simulink model "CAR_CONTROL_SYSTEM"  (R2024b)
settings: Solver=FixedStepAuto  StartTime=0.0  StopTime=inf  FixedStep=1e-3  RelTol=1e-3  EnableMultiTasking=on
model workspace (MAT data in the model file):
  SL_ROS_VariableLengthArrays_MaxSizes : object (value not decoded)
undefined symbols (not defined in the file or in its folder): angular, CIRCUIT, CLTF_DAMP, CLTF_FREQ, CLTF_GAIN, CONTROL, CONTROL_INI, DiscIntNeverNeededParam, dspblkCoreblockFVToolHelper, gcbh, INPUT, linear, MCP3201, MD25, MODEL, MODEL_INI, mpcstate, MPU60X0, MPU9250, MSG, NAV_MPC_CONTROL, OUTPUT, SAMPLING_TIME, SYSID_INPUT, VL6180X
libraries: raspberrypiCommlib x153, simulink x85, raspberrypiNetworklib x8, embedlinuxBasiclib x6, ctrlSharedLib x2, ros2lib x2, mpclib x1, vrlib x1, sldrtlib x1
(part 2 of 16)

== system CAR_CONTROL_SYSTEM/HARDWARE/COMMUNICATIONS ==
  MCS_RX : Subsystem  Commented=on  TreatAsAtomicUnit=on
      settings: MinAlgLoopOccurrences=on
  TCP/IP : Subsystem  TreatAsAtomicUnit=on
      settings: MinAlgLoopOccurrences=on
  TCP/IP RPI4 : Subsystem  TreatAsAtomicUnit=on
      settings: MinAlgLoopOccurrences=on

== system CAR_CONTROL_SYSTEM/HARDWARE/SENSORS ==
  BUTTONS : Subsystem  TreatAsAtomicUnit=on
      settings: MinAlgLoopOccurrences=on
  CURRENT_ADC_MCP3201_SPI : Subsystem  Commented=on  TreatAsAtomicUnit=on
      settings: RTWSystemCode=Nonreusable function  FunctionWithSeparateData=on
  IMU MPU60X0_SPI : Subsystem  Priority=0  TreatAsAtomicUnit=on
      settings: MinAlgLoopOccurrences=on  RTWSystemCode=Nonreusable function  FunctionWithSeparateData=on
  RCRX iBUS : Subsystem  TreatAsAtomicUnit=on
      settings: MinAlgLoopOccurrences=on
  WALL RANGE SENSOR : Subsystem
      settings: MinAlgLoopOccurrences=on

== system CAR_CONTROL_SYSTEM/MONITORING/BLACKBOX ==
  Compare To Constant : simulink/Logic and Bit Operations/Compare To Constant  relop===  const=uint8(2)  OutDataTypeStr=boolean
  Compare To Constant1 : simulink/Logic and Bit Operations/Compare To Constant  relop=>  const=uint8(2)  OutDataTypeStr=boolean
  Compare To Constant2 : simulink/Logic and Bit Operations/Compare To Constant  relop=~=  const=uint8(11)  OutDataTypeStr=boolean
  Data Store Read9 : DataStoreRead  DataStoreName=CONTROL  SampleTime=SAMPLING_TIME  DataStoreElements=CONTROL.STATE.COMM_MODE#CONTROL.STATE.CURRENT_STATUS_SYS  IndexOptions=Index vector (dialog)  Indices=1  OutputSizes=1
  HARDWARE: BLACKBOX : Subsystem  Priority=1000
  Logical Operator : Logic  Inputs=3  AllPortsSameDT=off  OutDataTypeStr=boolean
  PC: BLACKBOX : Subsystem
  wires:
  Data Store Read9/1 -> Compare To Constant/1
  Data Store Read9/2 -> Compare To Constant2/1, Compare To Constant1/1
  Compare To Constant/1 -> Logical Operator/1
  Compare To Constant1/1 -> Logical Operator/2
  Compare To Constant2/1 -> Logical Operator/3
  Logical Operator/1 -> HARDWARE: BLACKBOX/Enable, PC: BLACKBOX/Enable

== system CAR_CONTROL_SYSTEM/MONITORING/COMMUNICATIONS ==
  Compare To Zero1 : simulink/Logic and Bit Operations/Compare To Zero  relop=>  OutDataTypeStr=boolean
  Compare To Zero2 : simulink/Logic and Bit Operations/Compare To Zero  relop=>  OutDataTypeStr=boolean
  Data Store Read1 : DataStoreRead  DataStoreName=MSG  SampleTime=CONTROL_INI.PARAM.COMM_SAMPLING_TIME  DataStoreElements=MSG.RX_BUFFER(1,1)  IndexOptions=Index vector (dialog)  Indices=1  OutputSizes=1
  Data Store Read3 : DataStoreRead  DataStoreName=MSG  SampleTime=CONTROL_INI.PARAM.COMM_SAMPLING_TIME  DataStoreElements=MSG.TX_ID(1,1)  IndexOptions=Index vector (dialog)  Indices=1  OutputSizes=1
  MSG_RX : Subsystem  Priority=10
      settings: RTWSystemCode=Nonreusable function  FunctionWithSeparateData=on
  "MSG_TX " : Subsystem  Priority=10
      settings: RTWSystemCode=Nonreusable function  FunctionWithSeparateData=on
  wires:
  Data Store Read3/1 -> Compare To Zero2/1
  Compare To Zero2/1 -> "MSG_TX "/Enable
  Data Store Read1/1 -> Compare To Zero1/1
  Compare To Zero1/1 -> MSG_RX/Enable

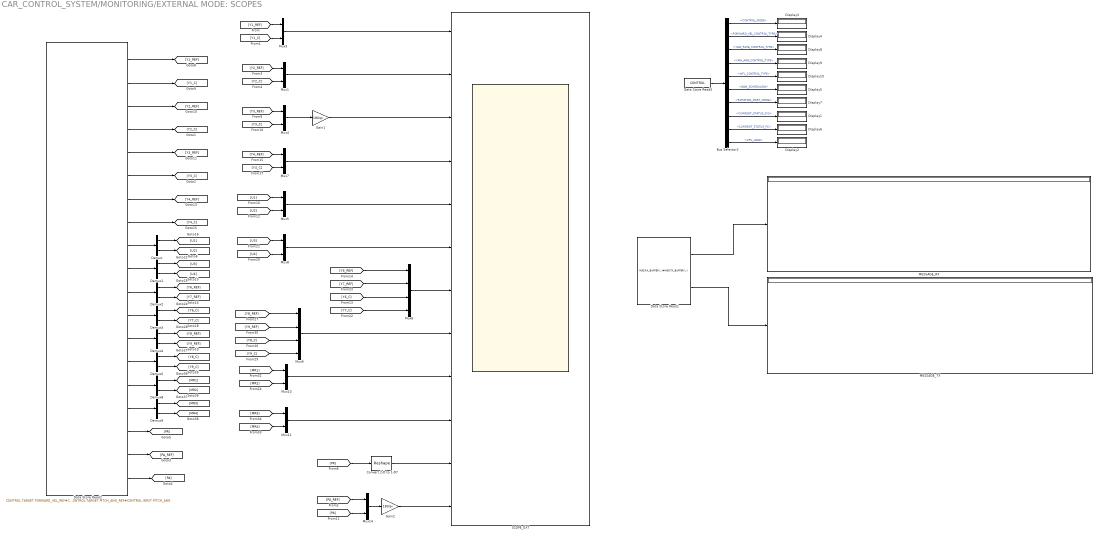
== system CAR_CONTROL_SYSTEM/MONITORING/EXTERNAL MODE: SCOPES ==
  Bus Selector2 : BusSelector  OutputSignals=STATE.CONTROL_MODE,STATE.FORWARD_VEL_CONTROL_TYPE,STATE.YAW_RATE_CONTROL_TYPE,STATE.YAW_ANG_CONTROL_TYPE,STATE.WFL_CONTROL_TYPE,STATE.GAIN_SCHEDULING,STATE.ROTATION_MSRT_MODE,STATE.CURRENT_STATUS_SYS,STATE.CURRENT_STATUS_PC,STATE.CPU_LOAD
  Convert 2-D to 1-D7 : Reshape
  Data Store Read1 : DataStoreRead  DataStoreName=MSG  SampleTime=SAMPLING_TIME  DataStoreElements=MSG.RX_BUFFER(:,:)#MSG.TX_BUFFER(:,:)  IndexOptions=Index vector (dialog)  Indices=1  OutputSizes=1
  Data Store Read2 : DataStoreRead  DataStoreName=CONTROL  SampleTime=SAMPLING_TIME  DataStoreElements=CONTROL.TARGET.FORWARD_VEL_REF#CONTROL.INPUT.FORWARD_VEL#CONTROL.TARGET.YAW_RATE_REF#CONTROL.INPUT.YAW_RATE#CONTROL.TARGET.YAW_ANG_REF#CONTROL.INPUT.YAW_ANG#CONTROL.TARGET.WALL_DIST_REF#CONTROL.INPUT.WALL_DIST#CONTROL.OUTPUT.MOTOR_VOLT(:,:)#CONTROL.OUTPUT.MOTOR_VOLT_CD(:,:)#CONTROL.TARGET.POS_XY_REF(:,:)#CONTROL.INPUT.EARTH_POS(1:2,1)#CONTROL.TARGET.VEL_XY_REF(:,:)#CONTROL.INPUT.EARTH_VEL(1:2,1)#CONTROL.INPUT.MOTOR_RATE(:,:)#CONTROL.INPUT.MOTOR_RATE_CD(:,:)#CONTROL.INPUT.PITCH_RATE#CONTROL.TARGET.PITCH_ANG_REF#CONTROL.INPUT.PITCH_ANG  IndexOptions=Index vector (dialog)  Indices=1  OutputSizes=1
  Data Store Read5 : DataStoreRead  DataStoreName=CONTROL  SampleTime=SAMPLING_TIME  IndexOptions=Index vector (dialog)  Indices=1  OutputSizes=1
  Demux{,1..5,8..9} (8 alike) : Demux  Outputs=2
  Display{1..10} (10 alike) : Display
  Gain1 : Gain  Gain=180/pi
  Gain2 : Gain  Gain=180/pi
  MESSAGE_RX : Display
  MESSAGE_TX : Display
  Mux{1,3..5,7..8,10..11,14} (9 alike) : Mux  Inputs=2
  Mux6 : Mux
  Mux9 : Mux
  SCOPE_EXT : Scope  NumInputPorts=12
  wires:
  Data Store Read5/1 -> Bus Selector2/1
  Bus Selector2/7 -> Display7/1  "<ROTATION_MSRT_MODE>"
  Data Store Read1/1 -> MESSAGE_RX/1
  Bus Selector2/2 -> Display4/1  "<FORWARD_VEL_CONTROL_TYPE>"
  Bus Selector2/1 -> Display3/1  "<CONTROL_MODE>"
  Bus Selector2/6 -> Display5/1  "<GAIN_SCHEDULING>"
  Bus Selector2/8 -> Display1/1  "<CURRENT_STATUS_SYS>"
  Bus Selector2/10 -> Display2/1  "<CPU_LOAD>"
  Data Store Read1/2 -> MESSAGE_TX/1
  Bus Selector2/9 -> Display6/1  "<CURRENT_STATUS_PC>"
  Demux8/2 -> [MR2]
  Demux9/1 -> [MR3]
  Data Store Read2/16 -> Demux9/1
  Data Store Read2/15 -> Demux8/1
  Data Store Read2/2 -> [Y1_C]
  Data Store Read2/7 -> [Y4_REF]
  Demux4/1 -> [Y8_REF]
  Demux5/1 -> [Y8_C]
  Demux3/1 -> [Y6_C]
  Demux2/1 -> [Y6_REF]
  Demux1/1 -> [U3]
  Demux3/2 -> [Y7_C]
  Demux5/2 -> [Y9_C]
  Demux4/2 -> [Y9_REF]
  Demux2/2 -> [Y7_REF]
  Data Store Read2/5 -> [Y3_REF]
  Demux/2 -> [U2]
  Data Store Read2/1 -> [Y1_REF]
  Demux1/2 -> [U4]
  Demux8/1 -> [MR1]
  Data Store Read2/4 -> [Y2_C]
  Data Store Read2/6 -> [Y3_C]
  Demux9/2 -> [MR4]
  Data Store Read2/3 -> [Y2_REF]
  Data Store Read2/8 -> [Y4_C]
  Demux/1 -> [U1]
  [MR1] -> Mux10/1
  [MR4] -> Mux11/2
  Gain1/1 -> SCOPE_EXT/3
  Mux10/1 -> SCOPE_EXT/9
  Mux8/1 -> SCOPE_EXT/6
  Mux6/1 -> SCOPE_EXT/7
  Mux5/1 -> SCOPE_EXT/5
  Mux7/1 -> SCOPE_EXT/4
  [MR3] -> Mux11/1
  [U4] -> Mux8/2
  Mux11/1 -> SCOPE_EXT/10
  [Y8_REF] -> Mux9/1
  [Y4_REF] -> Mux7/1
  [Y3_C] -> Mux4/2
  [Y4_C] -> Mux7/2
  [U1] -> Mux5/1
  Mux9/1 -> SCOPE_EXT/8
  [Y1_C] -> Mux3/2
  [U3] -> Mux8/1
  [U2] -> Mux5/2
  [Y2_C] -> Mux1/2
  [Y2_REF] -> Mux1/1
  Mux3/1 -> SCOPE_EXT/1
  [Y1_REF] -> Mux3/1
  [MR2] -> Mux10/2
  Mux4/1 -> Gain1/1
  Mux1/1 -> SCOPE_EXT/2
  [Y3_REF] -> Mux4/1
  [Y6_REF] -> Mux6/1
  [Y9_C] -> Mux9/4
  [Y7_C] -> Mux6/4
  Data Store Read2/9 -> Demux/1
  Data Store Read2/10 -> Demux1/1
  Data Store Read2/11 -> Demux2/1
  Data Store Read2/12 -> Demux3/1
  Data Store Read2/13 -> Demux4/1
  Data Store Read2/14 -> Demux5/1
  Bus Selector2/3 -> Display8/1  "<YAW_RATE_CONTROL_TYPE>"
  Bus Selector2/4 -> Display9/1  "<YAW_ANG_CONTROL_TYPE>"
  Bus Selector2/5 -> Display10/1  "<WFL_CONTROL_TYPE>"
  Data Store Read2/19 -> [PA]
  Data Store Read2/18 -> [PA_REF]
  Data Store Read2/17 -> [PR]
  [PA_REF] -> Mux14/1
  [PA] -> Mux14/2
  Mux14/1 -> Gain2/1
  Gain2/1 -> SCOPE_EXT/12
  [PR] -> Convert 2-D to 1-D7/1
  [Y6_C] -> Mux6/3
  [Y7_REF] -> Mux6/2
  [Y9_REF] -> Mux9/2
  [Y8_C] -> Mux9/3
  Convert 2-D to 1-D7/1 -> SCOPE_EXT/11

== system CAR_CONTROL_SYSTEM/MONITORING/FV COMPETITION: SCOPES ==
  Data Store Read1 : DataStoreRead  DataStoreName=CONTROL  SampleTime=SAMPLING_TIME  DataStoreElements=CONTROL.TARGET.FORWARD_VEL_REF#CONTROL.INPUT.FORWARD_VEL#CONTROL.OUTPUT.MOTOR_VOLT_CD(1,1)#CONTROL.STATE.COMP_IAE  IndexOptions=Index vector (dialog)  Indices=1  OutputSizes=1
  Display : Display
  FV COMPETITION SCOPE: SIM : Scope  NumInputPorts=3
  Mux6 : Mux  Inputs=2
  wires:
  Mux6/1 -> FV COMPETITION SCOPE: SIM/1
  Data Store Read1/1 -> Mux6/1
  Data Store Read1/2 -> Mux6/2
  Data Store Read1/3 -> FV COMPETITION SCOPE: SIM/2
  Data Store Read1/4 -> Display/1, FV COMPETITION SCOPE: SIM/3

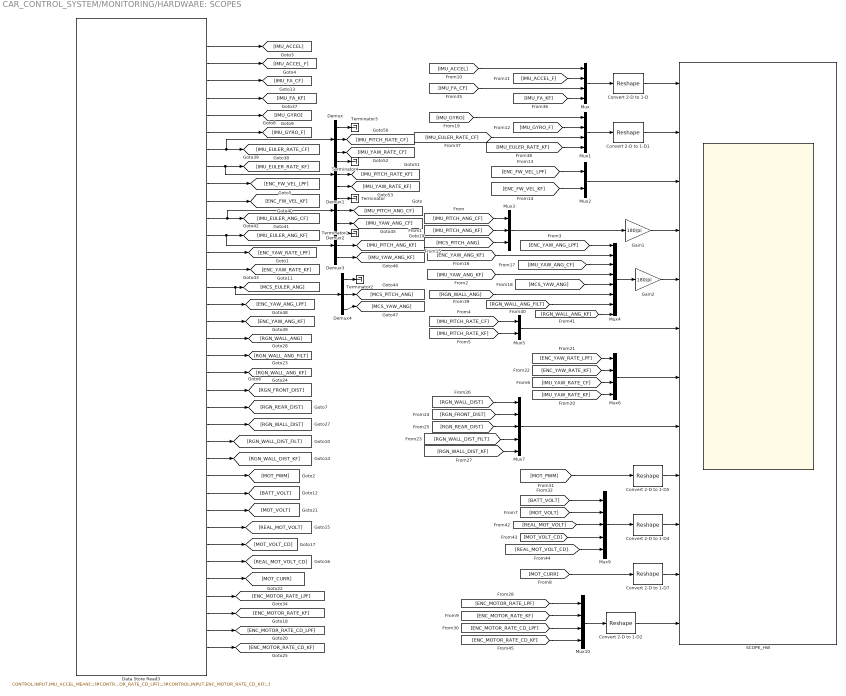
== system CAR_CONTROL_SYSTEM/MONITORING/HARDWARE: SCOPES ==
  Convert 2-D to 1-D{,1..2,4..5,7} (6 alike) : Reshape
  Data Store Read3 : DataStoreRead  DataStoreName=CONTROL  SampleTime=SAMPLING_TIME  DataStoreElements=CONTROL.INPUT.IMU_ACCEL_MEAN(:,:)#CONTROL.INPUT.IMU_ACCEL_MEAN_FILT(:,:)#CONTROL.INPUT.IMU_FORWARD_ACCEL_CF#CONTROL.INPUT.IMU_FORWARD_ACCEL_KF#CONTROL.INPUT.IMU_GYRO_MEAN(:,:)#CONTROL.INPUT.IMU_GYRO_MEAN_FILT(:,:)#CONTROL.INPUT.IMU_EULER_RATE_CF(:,:)#CONTROL.INPUT.IMU_EULER_RATE_KF(:,:)#CONTROL.INPUT.ENC_FORWARD_VEL_LPF#CONTROL.INPUT.ENC_FORWARD_VEL_KF#CONTROL.INPUT.IMU_EULER_ANG_CF(:,:)#CONTROL.INPUT.IMU_EULER_ANG_KF(:,:)#CONTROL.INPUT.ENC_YAW_RATE_LPF#CONTROL.INPUT.ENC_YAW_RATE_KF#CONTROL.INPUT.MCS_EULER_ANG(:,:)#CONTROL.INPUT.ENC_YAW_ANG_LPF#CONTROL.INPUT.ENC_YAW_ANG_KF#CONTROL.INPUT.RANGE_WALL_ANG#CONTROL.INPUT.WALL_ANG_FILT#CONTROL.INPUT.WALL_ANG_KF#CONTROL.INPUT.RANGE_FRONT_DIST#CONTROL.INPUT.RANGE_REAR_DIST#CONTROL.INPUT.RANGE_WALL_DIST#CONTROL.INPUT.WALL_DIST_FILT#CONTROL.INPUT.WALL_DIST_KF#CONTROL.OUTPUT.MOTOR_PWM(:,:)#CONTROL.INPUT.BATTERY_VOLT#CONTROL.OUTPUT.MOTOR_VOLT(:,:)#CONTROL.OUTPUT.REAL_MOTOR_VOLT(:,:)#CONTROL.OUTPUT.MOTOR_VOLT_CD(:,:)#CONTROL.OUTPUT.REAL_MOTOR_VOLT_CD(:,:)#CONTROL.INPUT.MOTOR_CURRENT(:,:)#CONTROL.INPUT.ENC_MOTOR_RATE_LPF(:,:)#CONTROL.INPUT.ENC_MOTOR_RATE_KF(:,:)#CONTROL.INPUT.ENC_MOTOR_RATE_CD_LPF(:,:)#CONTROL.INPUT.ENC_MOTOR_RATE_CD_KF(:,:)  IndexOptions=Index vector (dialog)  Indices=1  OutputSizes=1
  Demux{,1..4} (5 alike) : Demux  Outputs=3
  Gain1 : Gain  Gain=180/pi
  Gain2 : Gain  Gain=180/pi
  Mux{,1,6,10} (4 alike) : Mux
  Mux2 : Mux  Inputs=2
  Mux3 : Mux  Inputs=3
  Mux4 : Mux  Inputs=8
  Mux5 : Mux  Inputs=2
  Mux7 : Mux  Inputs=5
  Mux9 : Mux  Inputs=5
  SCOPE_HW : Scope  NumInputPorts=12
  Terminator{,1..4} (5 alike) : Terminator
  wires:
  [MOT_CURR] -> Convert 2-D to 1-D7/1
  Convert 2-D to 1-D/1 -> SCOPE_HW/1
  Convert 2-D to 1-D1/1 -> SCOPE_HW/2
  Mux2/1 -> SCOPE_HW/3
  [IMU_ACCEL] -> Mux/1
  Mux/1 -> Convert 2-D to 1-D/1
  [IMU_ACCEL_F] -> Mux/2
  [ENC_FW_VEL_LPF] -> Mux2/1
  [ENC_FW_VEL_KF] -> Mux2/2
  [IMU_PITCH_ANG_CF] -> Mux3/1
  [IMU_PITCH_ANG_KF] -> Mux3/2
  Mux3/1 -> Gain1/1
  Gain1/1 -> SCOPE_HW/4
  Mux4/1 -> Gain2/1
  Gain2/1 -> SCOPE_HW/5
  Mux5/1 -> SCOPE_HW/6
  [IMU_PITCH_RATE_CF] -> Mux5/1
  [IMU_PITCH_RATE_KF] -> Mux5/2
  Mux6/1 -> SCOPE_HW/7
  Mux7/1 -> SCOPE_HW/8
  [RGN_WALL_DIST] -> Mux7/1
  [RGN_FRONT_DIST] -> Mux7/2
  [RGN_REAR_DIST] -> Mux7/3
  Mux9/1 -> Convert 2-D to 1-D4/1
  [MOT_VOLT] -> Mux9/2
  [BATT_VOLT] -> Mux9/1
  [MOT_PWM] -> Convert 2-D to 1-D5/1
  Convert 2-D to 1-D5/1 -> SCOPE_HW/9
  Convert 2-D to 1-D4/1 -> SCOPE_HW/10
  Convert 2-D to 1-D7/1 -> SCOPE_HW/11
  Data Store Read3/1 -> [IMU_ACCEL]
  Data Store Read3/2 -> [IMU_ACCEL_F]
  [ENC_MOTOR_RATE_KF] -> Mux10/2
  Mux10/1 -> Convert 2-D to 1-D2/1
  [ENC_MOTOR_RATE_LPF] -> Mux10/1
  Data Store Read3/32 -> [MOT_CURR]
  Data Store Read3/33 -> [ENC_MOTOR_RATE_LPF]
  Data Store Read3/34 -> [ENC_MOTOR_RATE_KF]
  Data Store Read3/5 -> [IMU_GYRO]
  Data Store Read3/6 -> [IMU_GYRO_F]
  Data Store Read3/3 -> [IMU_FA_CF]
  Data Store Read3/4 -> [IMU_FA_KF]
  [IMU_FA_CF] -> Mux/3
  [IMU_FA_KF] -> Mux/4
  Data Store Read3/7 -> Demux/1, [IMU_EULER_RATE_CF]
  Data Store Read3/8 -> Demux1/1, [IMU_EULER_RATE_KF]
  Mux1/1 -> Convert 2-D to 1-D1/1
  [IMU_GYRO] -> Mux1/1
  [IMU_GYRO_F] -> Mux1/2
  [IMU_EULER_RATE_CF] -> Mux1/3
  [IMU_EULER_RATE_KF] -> Mux1/4
  Data Store Read3/9 -> [ENC_FW_VEL_LPF]
  Data Store Read3/10 -> [ENC_FW_VEL_KF]
  Data Store Read3/11 -> Demux2/1, [IMU_EULER_ANG_CF]
  Data Store Read3/12 -> Demux3/1, [IMU_EULER_ANG_KF]
  Demux2/2 -> [IMU_PITCH_ANG_CF]
  Demux3/2 -> [IMU_PITCH_ANG_KF]
  Demux4/2 -> [MCS_PITCH_ANG]
  [MCS_PITCH_ANG] -> Mux3/3
  Demux2/3 -> [IMU_YAW_ANG_CF]
  Demux3/3 -> [IMU_YAW_ANG_KF]
  Demux2/1 -> Terminator/1
  Demux3/1 -> Terminator1/1
  Demux4/3 -> [MCS_YAW_ANG]
  Demux4/1 -> Terminator2/1
  [ENC_YAW_ANG_LPF] -> Mux4/1
  [ENC_YAW_ANG_KF] -> Mux4/2
  [IMU_YAW_ANG_CF] -> Mux4/3
  [IMU_YAW_ANG_KF] -> Mux4/4
  [MCS_YAW_ANG] -> Mux4/5
  [RGN_WALL_ANG] -> Mux4/6
  [RGN_WALL_ANG_FILT] -> Mux4/7
  [RGN_WALL_ANG_KF] -> Mux4/8
  Demux/2 -> [IMU_PITCH_RATE_CF]
  Demux1/2 -> [IMU_PITCH_RATE_KF]
  Demux/1 -> Terminator3/1
  Demux1/1 -> Terminator4/1
  Demux/3 -> [IMU_YAW_RATE_CF]
  Demux1/3 -> [IMU_YAW_RATE_KF]
  Data Store Read3/14 -> [ENC_YAW_RATE_KF]
  Data Store Read3/15 -> Demux4/1, [MCS_EULER_ANG]
  Data Store Read3/16 -> [ENC_YAW_ANG_LPF]
  Data Store Read3/17 -> [ENC_YAW_ANG_KF]
  Data Store Read3/18 -> [RGN_WALL_ANG]
  Data Store Read3/19 -> [RGN_WALL_ANG_FILT]
  Data Store Read3/20 -> [RGN_WALL_ANG_KF]
  Data Store Read3/13 -> [ENC_YAW_RATE_LPF]
  Data Store Read3/21 -> [RGN_FRONT_DIST]
  Data Store Read3/22 -> [RGN_REAR_DIST]
  Data Store Read3/23 -> [RGN_WALL_DIST]
  Data Store Read3/24 -> [RGN_WALL_DIST_FILT]
  Data Store Read3/25 -> [RGN_WALL_DIST_KF]
  [RGN_WALL_DIST_FILT] -> Mux7/4
  [RGN_WALL_DIST_KF] -> Mux7/5
  Data Store Read3/26 -> [MOT_PWM]
  Data Store Read3/27 -> [BATT_VOLT]
  Data Store Read3/28 -> [MOT_VOLT]
  Data Store Read3/29 -> [REAL_MOT_VOLT]
  Data Store Read3/31 -> [REAL_MOT_VOLT_CD]
  Data Store Read3/30 -> [MOT_VOLT_CD]
  [REAL_MOT_VOLT_CD] -> Mux9/5
  [REAL_MOT_VOLT] -> Mux9/3
  [MOT_VOLT_CD] -> Mux9/4
  Data Store Read3/35 -> [ENC_MOTOR_RATE_CD_LPF]
  Data Store Read3/36 -> [ENC_MOTOR_RATE_CD_KF]
  [ENC_MOTOR_RATE_CD_LPF] -> Mux10/3
  [ENC_MOTOR_RATE_CD_KF] -> Mux10/4
  Convert 2-D to 1-D2/1 -> SCOPE_HW/12
  [IMU_YAW_RATE_CF] -> Mux6/3
  [IMU_YAW_RATE_KF] -> Mux6/4
  [ENC_YAW_RATE_LPF] -> Mux6/1
  [ENC_YAW_RATE_KF] -> Mux6/2

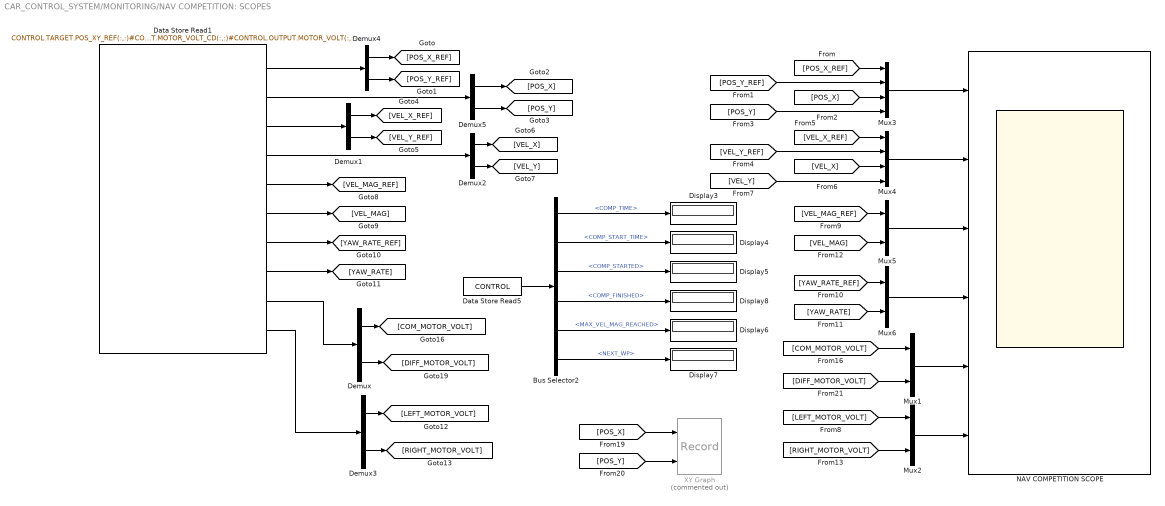
== system CAR_CONTROL_SYSTEM/MONITORING/NAV COMPETITION: SCOPES ==
  Bus Selector2 : BusSelector  OutputSignals=STATE.COMP_TIME,STATE.COMP_START_TIME,STATE.COMP_STARTED,STATE.COMP_FINISHED,STATE.MAX_VEL_MAG_REACHED,STATE.NEXT_WP
  Data Store Read1 : DataStoreRead  DataStoreName=CONTROL  SampleTime=SAMPLING_TIME  DataStoreElements=CONTROL.TARGET.POS_XY_REF(:,:)#CONTROL.INPUT.EARTH_POS(1:2,1)#CONTROL.TARGET.VEL_XY_REF(:,:)#CONTROL.INPUT.EARTH_VEL(1:2,1)#CONTROL.TARGET.FORWARD_VEL_REF#CONTROL.INPUT.FORWARD_VEL#CONTROL.TARGET.YAW_RATE_REF#CONTROL.INPUT.YAW_RATE#CONTROL.OUTPUT.MOTOR_VOLT_CD(:,:)#CONTROL.OUTPUT.MOTOR_VOLT(:,:)  IndexOptions=Index vector (dialog)  Indices=1  OutputSizes=1
  Data Store Read5 : DataStoreRead  DataStoreName=CONTROL  SampleTime=SAMPLING_TIME  IndexOptions=Index vector (dialog)  Indices=1  OutputSizes=1
  Demux{,1..5} (6 alike) : Demux  Outputs=2
  Display{3..8} (6 alike) : Display
  Mux{1..2,5..6} (4 alike) : Mux  Inputs=2
  Mux3 : Mux
  Mux4 : Mux
  NAV COMPETITION SCOPE : Scope  NumInputPorts=6
  XY Graph : Record  Commented=on  FileSettingsInternal="{\"entries\":[{\"content\":{\"excelSettings\":{\"content\":{},\"type\":\"Streamout.ExcelSettings\"}},\"type\":\"Streamout.FileSettingStorage\",\"uuid\":\"\"}],\"packageUris\":[\"http:\\/\\/schema.mathworks.com\\/mf0\\/streamout_blocks\\/R2020a\"],\"version\":\"1.0\"}"  Layout=[1 1]  SignalsInternal="{\"entries\":[{\"content\":{\"signals\":[{\"content\":{\"blockPath\":[],\"dimensions\":[1],\"domain\":\"\",\"lineColor\":\"#a2142f\",\"plots\":[ 1 ],\"port\":1,\"signalID\":1,\"signalName\":\"XY Graph:1\"},\"type\":\"RecordBlkView.Signal\",\"uuid\":\"\"},{\"content\":{\"blockPath\":[],\"dimensions\":[1],\"domain\":\"\",\"lineColor\":\"#139fff\",\"plots\":[ 1 ],\"port\":2,\"signalID\":2,\"signalName\":\"XY Graph:2\"},\"type\":\"RecordBlkView.Signal\",\"uuid\":\"\"}]},\"type\":\"RecordBlkView.InputSignals\",\"uuid\":\"\"}],\"packageUris\":[\"http:\\/\\/schema.mathworks.com\\/mf0\\/streamout_blocks\\/R2020a\"],\"version\":\"1.0\"}"  VisualizationBindings="{\"xyplotplugin\":{\"info\":[{\"series\":[{\"bindingParametersList\":[{\"parameter\":\"X-Axis\",\"signalID\":1,\"signalName\":\"XY Graph:1\"},{\"parameter\":\"Y-Axis\",\"signalID\":2,\"signalName\":\"XY Graph:2\"}],\"seriesID\":0}],\"subplotID\":1}]}}"  CompatibilityTag=XY  st=SAMPLING_TIME
  wires:
  Bus Selector2/1 -> Display3/1  "<COMP_TIME>"
  Bus Selector2/4 -> Display8/1  "<COMP_FINISHED>"
  Bus Selector2/3 -> Display5/1  "<COMP_STARTED>"
  Bus Selector2/2 -> Display4/1  "<COMP_START_TIME>"
  Bus Selector2/6 -> Display7/1  "<NEXT_WP>"
  Mux4/1 -> NAV COMPETITION SCOPE/2
  Bus Selector2/5 -> Display6/1  "<MAX_VEL_MAG_REACHED>"
  Mux6/1 -> NAV COMPETITION SCOPE/4
  Mux3/1 -> NAV COMPETITION SCOPE/1
  Mux5/1 -> NAV COMPETITION SCOPE/3
  Data Store Read5/1 -> Bus Selector2/1
  Demux4/1 -> [POS_X_REF]
  Demux4/2 -> [POS_Y_REF]
  Demux5/1 -> [POS_X]
  Demux5/2 -> [POS_Y]
  [POS_X_REF] -> Mux3/1
  [VEL_X_REF] -> Mux4/1
  [VEL_Y] -> Mux4/4
  [VEL_MAG_REF] -> Mux5/1
  [VEL_MAG] -> Mux5/2
  [YAW_RATE_REF] -> Mux6/1
  [YAW_RATE] -> Mux6/2
  Data Store Read1/9 -> Demux/1
  [POS_X] -> XY Graph/1
  [POS_Y] -> XY Graph/2
  Demux1/1 -> [VEL_X_REF]
  Demux1/2 -> [VEL_Y_REF]
  Demux2/2 -> [VEL_Y]
  Demux2/1 -> [VEL_X]
  Data Store Read1/1 -> Demux4/1
  Data Store Read1/2 -> Demux5/1
  Data Store Read1/3 -> Demux1/1
  Data Store Read1/4 -> Demux2/1
  Data Store Read1/5 -> [VEL_MAG_REF]
  Data Store Read1/6 -> [VEL_MAG]
  Data Store Read1/7 -> [YAW_RATE_REF]
  Data Store Read1/8 -> [YAW_RATE]
  Demux/1 -> [COM_MOTOR_VOLT]
  Demux/2 -> [DIFF_MOTOR_VOLT]
  [COM_MOTOR_VOLT] -> Mux1/1
  [DIFF_MOTOR_VOLT] -> Mux1/2
  Mux1/1 -> NAV COMPETITION SCOPE/5
  Mux2/1 -> NAV COMPETITION SCOPE/6
  [RIGHT_MOTOR_VOLT] -> Mux2/2
  [LEFT_MOTOR_VOLT] -> Mux2/1
  Data Store Read1/10 -> Demux3/1
  Demux3/1 -> [LEFT_MOTOR_VOLT]
  Demux3/2 -> [RIGHT_MOTOR_VOLT]
  [POS_Y_REF] -> Mux3/2
  [POS_X] -> Mux3/3
  [POS_Y] -> Mux3/4
  [VEL_Y_REF] -> Mux4/2
  [VEL_X] -> Mux4/3

== system CAR_CONTROL_SYSTEM/MONITORING/ROS_COM ==
  note: ESTE BLOQUE SE USO PARA HACER UN CONTROL DE VELOCIDAD RENDERIZADO EN
      | GAZEBO CON SIMULACION FISICA EN SIMULINK.
  Constant : Constant  Value=-0.25  SampleTime=SAMPLING_TIME
  Constant1 : Constant  Value=-0.25  SampleTime=SAMPLING_TIME
  DYNAMICS PUBLISHERS : Subsystem
  Data Store Write : DataStoreWrite  DataStoreName=CONTROL  DataStoreElements=CONTROL.TARGET.NAV_REF_PC(:,:)  IndexOptions=Index vector (dialog)  Indices=1  OutputSizes=1
  Mux : Mux  Inputs=2
  wires:
  Mux/1 -> Data Store Write/1
  Constant/1 -> Mux/1
  Constant1/1 -> Mux/2

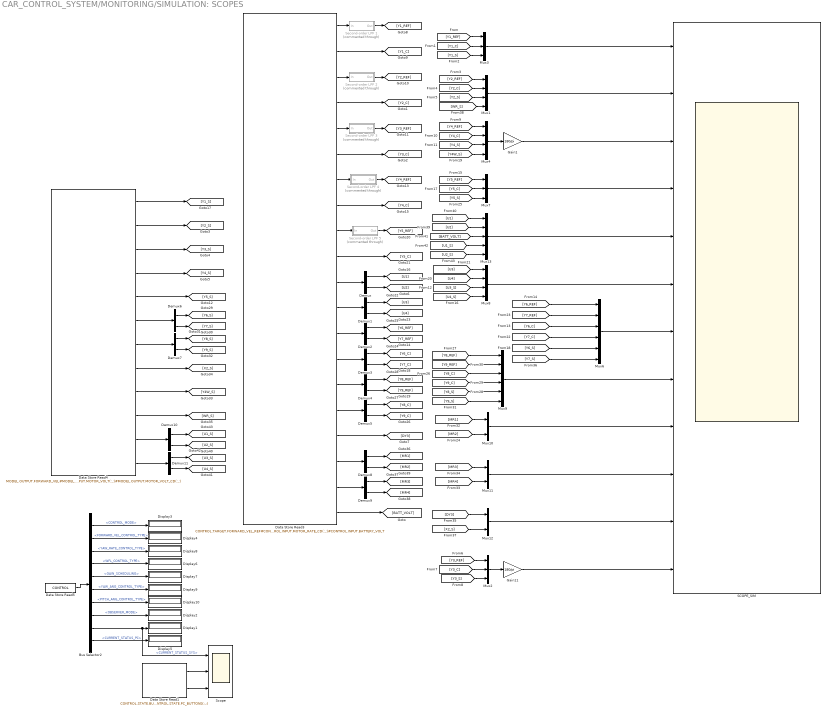
== system CAR_CONTROL_SYSTEM/MONITORING/SIMULATION: SCOPES ==
  Bus Selector2 : BusSelector  OutputSignals=STATE.CONTROL_MODE,STATE.FORWARD_VEL_CONTROL_TYPE,STATE.YAW_RATE_CONTROL_TYPE,STATE.WFL_CONTROL_TYPE,STATE.GAIN_SCHEDULING,STATE.YAW_ANG_CONTROL_TYPE,STATE.PITCH_ANG_CONTROL_TYPE,STATE.OBSERVER_MODE,STATE.CURRENT_STATUS_SYS,STATE.CURRENT_STATUS_PC
  Data Store Read1 : DataStoreRead  DataStoreName=CONTROL  SampleTime=SAMPLING_TIME  DataStoreElements=CONTROL.STATE.BUTTONS(:,:)#CONTROL.STATE.PC_BUTTONS(:,:)  IndexOptions=Index vector (dialog)  Indices=1  OutputSizes=1
  Data Store Read3 : DataStoreRead  DataStoreName=CONTROL  SampleTime=SAMPLING_TIME  DataStoreElements=CONTROL.TARGET.FORWARD_VEL_REF#CONTROL.INPUT.FORWARD_VEL#CONTROL.TARGET.YAW_RATE_REF#CONTROL.INPUT.YAW_RATE#CONTROL.TARGET.PITCH_ANG_REF#CONTROL.INPUT.PITCH_ANG#CONTROL.TARGET.YAW_ANG_REF#CONTROL.INPUT.YAW_ANG#CONTROL.TARGET.WALL_DIST_REF#CONTROL.INPUT.WALL_DIST#CONTROL.OUTPUT.MOTOR_VOLT(:,:)#CONTROL.OUTPUT.MOTOR_VOLT_CD(:,:)#CONTROL.TARGET.POS_XY_REF(:,:)#CONTROL.INPUT.EARTH_POS(1:2,1)#CONTROL.TARGET.VEL_XY_REF(:,:)#CONTROL.INPUT.EARTH_VEL(1:2,1)#CONTROL.INPUT.PITCH_RATE#CONTROL.INPUT.MOTOR_RATE(:,:)#CONTROL.INPUT.MOTOR_RATE_CD(:,:)#CONTROL.INPUT.BATTERY_VOLT  IndexOptions=Index vector (dialog)  Indices=1  OutputSizes=1
  Data Store Read4 : DataStoreRead  DataStoreName=MODEL  SampleTime=SAMPLING_TIME  DataStoreElements=MODEL.OUTPUT.FORWARD_VEL#MODEL.OUTPUT.YAW_RATE#MODEL.OUTPUT.PITCH_ANG#MODEL.OUTPUT.YAW_ANG#MODEL.OUTPUT.WALL_DIST#MODEL.OUTPUT.EARTH_POS(1:2,1)#MODEL.OUTPUT.EARTH_VEL(1:2,1)#MODEL.OUTPUT.PITCH_RATE#MODEL.OUTPUT.WALL_ANG#MODEL.INPUT.WALL_RATE#MODEL.INPUT.MOTOR_VOLT(:,:)#MODEL.OUTPUT.MOTOR_VOLT_CD(:,:)  IndexOptions=Index vector (dialog)  Indices=1  OutputSizes=1
  Data Store Read5 : DataStoreRead  DataStoreName=CONTROL  SampleTime=SAMPLING_TIME  IndexOptions=Index vector (dialog)  Indices=1  OutputSizes=1
  Demux{,1..11} (12 alike) : Demux  Outputs=2
  Display{1..10} (10 alike) : Display
  Gain1 : Gain  Gain=180/pi
  Gain11 : Gain  Gain=180/pi
  Mux1 : Mux
  Mux10 : Mux  Inputs=2
  Mux11 : Mux  Inputs=2
  Mux12 : Mux  Inputs=2
  Mux13 : Mux  Inputs=5
  Mux2 : Mux  Inputs=3
  Mux3 : Mux  Inputs=3
  Mux4 : Mux
  Mux6 : Mux  Inputs=6
  Mux7 : Mux  Inputs=3
  Mux8 : Mux
  Mux9 : Mux  Inputs=6
  SCOPE_SIM : Scope  NumInputPorts=12
  Scope : Scope  NumInputPorts=3
  Second-order LPF 1 : Subsystem  Commented=through  mask{Fo=CLTF_GAIN(1), wn=CLTF_FREQ(1), seta=CLTF_DAMP(1), ts=SAMPLING_TIME}
      mask prompts: Fo "Static gain"; wn "Natural frequency (rad/s)"; seta "Damping factor"; ts "Sampling time"
      mask init:
      | s=tf('s');
      | F = Fo/(s^2/wn^2+2*seta/wn*s+1);
      | Fd = c2d(F,ts,'tustin');
      mask DialogControl LPF_PARAM Prompt: Filter parameters
  Second-order LPF 2 : Subsystem  Commented=through  mask{Fo=CLTF_GAIN(2), wn=CLTF_FREQ(2), seta=CLTF_DAMP(2), ts=SAMPLING_TIME}
      mask prompts: Fo "Static gain"; wn "Natural frequency (rad/s)"; seta "Damping factor"; ts "Sampling time"
      mask init:
      | s=tf('s');
      | F = Fo/(s^2/wn^2+2*seta/wn*s+1);
      | Fd = c2d(F,ts,'tustin');
      mask DialogControl LPF_PARAM Prompt: Filter parameters
  Second-order LPF 3 : Subsystem  Commented=through  mask{Fo=CLTF_GAIN(3), wn=CLTF_FREQ(3), seta=CLTF_DAMP(3), ts=SAMPLING_TIME}
      mask prompts: Fo "Static gain"; wn "Natural frequency (rad/s)"; seta "Damping factor"; ts "Sampling time"
      mask init:
      | s=tf('s');
      | F = Fo/(s^2/wn^2+2*seta/wn*s+1);
      | Fd = c2d(F,ts,'tustin');
      mask DialogControl LPF_PARAM Prompt: Filter parameters
  Second-order LPF 4 : Subsystem  Commented=through  mask{Fo=CLTF_GAIN(4), wn=CLTF_FREQ(4), seta=CLTF_DAMP(4), ts=SAMPLING_TIME}
      mask prompts: Fo "Static gain"; wn "Natural frequency (rad/s)"; seta "Damping factor"; ts "Sampling time"
      mask init:
      | s=tf('s');
      | F = Fo/(s^2/wn^2+2*seta/wn*s+1);
      | Fd = c2d(F,ts,'tustin');
      mask DialogControl LPF_PARAM Prompt: Filter parameters
  Second-order LPF 5 : Subsystem  Commented=through  mask{Fo=CLTF_GAIN(5), wn=CLTF_FREQ(5), seta=CLTF_DAMP(5), ts=SAMPLING_TIME}
      mask prompts: Fo "Static gain"; wn "Natural frequency (rad/s)"; seta "Damping factor"; ts "Sampling time"
      mask init:
      | s=tf('s');
      | F = Fo/(s^2/wn^2+2*seta/wn*s+1);
      | Fd = c2d(F,ts,'tustin');
      mask DialogControl LPF_PARAM Prompt: Filter parameters
  wires:
  Data Store Read3/2 -> [Y1_C]
  Data Store Read3/1 -> Second-order LPF 1/1(In)
  Mux3/1 -> SCOPE_SIM/1
  Mux1/1 -> SCOPE_SIM/2
  Data Store Read3/5 -> Second-order LPF 3/1(In)
  Data Store Read3/3 -> Second-order LPF 2/1(In)
  [Y2_REF] -> Mux1/1
  [Y4_REF] -> Mux4/1
  [Y1_REF] -> Mux3/1
  Data Store Read3/8 -> [Y4_C]
  Data Store Read3/4 -> [Y2_C]
  Mux4/1 -> Gain1/1
  Data Store Read3/7 -> Second-order LPF 4/1(In)
  Second-order LPF 1/1(Out) -> [Y1_REF]
  Second-order LPF 2/1(Out) -> [Y2_REF]
  Second-order LPF 3/1(Out) -> [Y3_REF]
  Second-order LPF 4/1(Out) -> [Y4_REF]
  Bus Selector2/1 -> Display3/1  "<CONTROL_MODE>"
  Data Store Read5/1 -> Bus Selector2/1
  Bus Selector2/2 -> Display4/1  "<FORWARD_VEL_CONTROL_TYPE>"
  Bus Selector2/5 -> Display7/1  "<GAIN_SCHEDULING>"
  Bus Selector2/9 -> Scope/1, Display1/1  "<CURRENT_STATUS_SYS>"
  [Y6_REF] -> Mux6/1
  Data Store Read3/6 -> [Y3_C]
  Bus Selector2/3 -> Display8/1  "<YAW_RATE_CONTROL_TYPE>"
  Bus Selector2/4 -> Display6/1  "<WFL_CONTROL_TYPE>"
  [Y1_C] -> Mux3/2
  [Y1_S] -> Mux3/3
  [Y2_S] -> Mux1/3
  [Y2_C] -> Mux1/2
  [Y4_S] -> Mux4/3
  [Y4_C] -> Mux4/2
  Data Store Read4/1 -> [Y1_S]
  Data Store Read4/2 -> [Y2_S]
  Data Store Read4/3 -> [Y3_S]
  Data Store Read4/4 -> [Y4_S]
  Second-order LPF 5/1(Out) -> [Y5_REF]
  Data Store Read3/10 -> [Y5_C]
  Data Store Read3/9 -> Second-order LPF 5/1(In)
  Data Store Read3/11 -> Demux/1
  Demux/1 -> [U1]
  Demux/2 -> [U2]
  Demux1/2 -> [U4]
  Demux1/1 -> [U3]
  Data Store Read3/12 -> Demux1/1
  Data Store Read3/13 -> Demux2/1
  Demux2/1 -> [Y6_REF]
  Demux2/2 -> [Y7_REF]
  Data Store Read3/14 -> Demux3/1
  Demux3/1 -> [Y6_C]
  Demux3/2 -> [Y7_C]
  Demux4/1 -> [Y8_REF]
  Demux4/2 -> [Y9_REF]
  Demux5/2 -> [Y9_C]
  Data Store Read3/16 -> Demux5/1
  Data Store Read3/15 -> Demux4/1
  Demux5/1 -> [Y8_C]
  Data Store Read4/5 -> [Y5_S]
  Data Store Read4/6 -> Demux6/1
  Demux6/1 -> [Y6_S]
  Demux6/2 -> [Y7_S]
  Demux7/2 -> [Y9_S]
  Demux7/1 -> [Y8_S]
  Data Store Read4/7 -> Demux7/1
  Data Store Read4/9 -> [Y4W_S]
  Data Store Read4/8 -> [X2_S]
  Data Store Read4/10 -> [WR_S]
  Bus Selector2/8 -> Display2/1  "<OBSERVER_MODE>"
  [Y4W_S] -> Mux4/4
  [Y5_C] -> Mux7/2
  [Y5_S] -> Mux7/3
  [Y5_REF] -> Mux7/1
  [Y9_S] -> Mux9/6
  Gain1/1 -> SCOPE_SIM/3
  Mux7/1 -> SCOPE_SIM/4
  Mux13/1 -> SCOPE_SIM/5
  Mux6/1 -> SCOPE_SIM/7
  Mux9/1 -> SCOPE_SIM/8
  Demux8/1 -> [MR1]
  Demux8/2 -> [MR2]
  Demux9/1 -> [MR3]
  Demux9/2 -> [MR4]
  Data Store Read3/17 -> [DY3]
  Data Store Read3/18 -> Demux8/1
  Data Store Read3/19 -> Demux9/1
  [Y8_REF] -> Mux9/1
  Gain11/1 -> SCOPE_SIM/12
  Mux2/1 -> Gain11/1
  [Y3_REF] -> Mux2/1
  Mux11/1 -> SCOPE_SIM/10
  [MR4] -> Mux11/2
  Mux10/1 -> SCOPE_SIM/9
  [MR1] -> Mux10/1
  [MR3] -> Mux11/1
  [MR2] -> Mux10/2
  Mux12/1 -> SCOPE_SIM/11
  Bus Selector2/10 -> Display5/1  "<CURRENT_STATUS_PC>"
  Data Store Read1/1 -> Scope/2
  Data Store Read1/2 -> Scope/3
  [Y7_S] -> Mux6/6
  [WR_S] -> Mux1/4
  Bus Selector2/6 -> Display9/1  "<YAW_ANG_CONTROL_TYPE>"
  Bus Selector2/7 -> Display10/1  "<PITCH_ANG_CONTROL_TYPE>"
  [U1] -> Mux13/1
  [U2] -> Mux13/2
  [U1_S] -> Mux13/4
  [U2_S] -> Mux13/5
  [BATT_VOLT] -> Mux13/3
  [U4] -> Mux8/2
  [U3] -> Mux8/1
  [U3_S] -> Mux8/3
  [U4_S] -> Mux8/4
  Mux8/1 -> SCOPE_SIM/6
  Data Store Read3/20 -> [BATT_VOLT]
  Demux10/1 -> [U1_S]
  Demux10/2 -> [U2_S]
  Data Store Read4/11 -> Demux10/1
  Demux11/1 -> [U3_S]
  Data Store Read4/12 -> Demux11/1
  Demux11/2 -> [U4_S]
  [Y3_S] -> Mux2/3
  [X2_S] -> Mux12/2
  [DY3] -> Mux12/1
  [Y3_C] -> Mux2/2
  [Y7_REF] -> Mux6/2
  [Y6_C] -> Mux6/3
  [Y7_C] -> Mux6/4
  [Y6_S] -> Mux6/5
  [Y9_REF] -> Mux9/2
  [Y8_C] -> Mux9/3
  [Y9_C] -> Mux9/4
  [Y8_S] -> Mux9/5

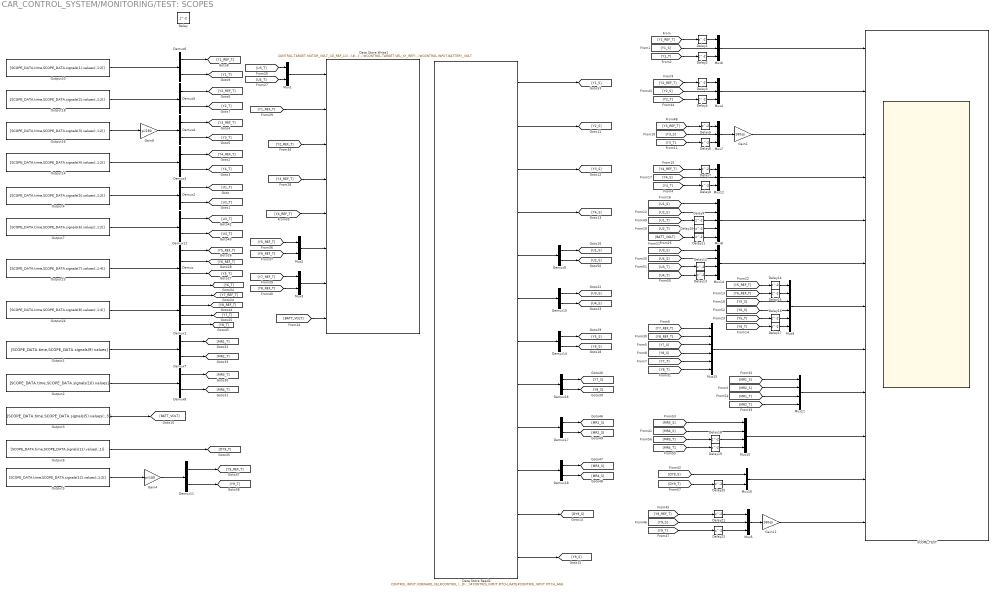
== system CAR_CONTROL_SYSTEM/MONITORING/TEST: SCOPES ==
  Data Store Read2 : DataStoreRead  DataStoreName=CONTROL  SampleTime=SAMPLING_TIME  DataStoreElements=CONTROL.INPUT.FORWARD_VEL#CONTROL.INPUT.YAW_RATE#CONTROL.INPUT.YAW_ANG#CONTROL.INPUT.WALL_DIST#CONTROL.OUTPUT.MOTOR_VOLT(:,:)#CONTROL.OUTPUT.MOTOR_VOLT_CD(:,:)#CONTROL.INPUT.EARTH_POS(1:2,1)#CONTROL.INPUT.EARTH_VEL(1:2,1)#CONTROL.INPUT.MOTOR_RATE(:,:)#CONTROL.INPUT.MOTOR_RATE_CD(:,:)#CONTROL.INPUT.PITCH_RATE#CONTROL.INPUT.PITCH_ANG  IndexOptions=Index vector (dialog)  Indices=1  OutputSizes=1
  Data Store Write1 : DataStoreWrite  DataStoreName=CONTROL  SampleTime=SAMPLING_TIME  DataStoreElements=CONTROL.TARGET.MOTOR_VOLT_CD_REF_LC(:,:)#CONTROL.TARGET.FORWARD_VEL_REF_LC#CONTROL.TARGET.YAW_RATE_REF_LC#CONTROL.TARGET.YAW_ANG_REF_LC#CONTROL.TARGET.WALL_DIST_REF_LC#CONTROL.TARGET.POS_XY_REF(:,:)#CONTROL.TARGET.VEL_XY_REF(:,:)#CONTROL.INPUT.BATTERY_VOLT  IndexOptions=Index vector (dialog)  Indices=1  OutputSizes=1
  Delay{,1..22} (23 alike) : Delay
  Demux : Demux
  Demux1 : Demux
  Demux{2..5,7..12,14,16..18} (14 alike) : Demux  Outputs=2
  Demux6 : Demux  Outputs=[1 1]
  Gain1 : Gain  Gain=180/pi
  Gain11 : Gain  Gain=180/pi
  Gain4 : Gain  Gain=pi/180
  Gain8 : Gain  Gain=pi/180
  Mux{1..3,16} (4 alike) : Mux  Inputs=2
  Mux10 : Mux
  Mux11 : Mux
  Mux{4..7,12} (5 alike) : Mux  Inputs=3
  Mux14 : Mux
  Mux15 : Mux  Inputs=6
  Mux8 : Mux  Inputs=5
  Mux9 : Mux  Inputs=6
  Output1 : FromWorkspace  VariableName=[SCOPE_DATA.time,SCOPE_DATA.signals(9).values]  SampleTime=SAMPLING_TIME
  Output14 : FromWorkspace  VariableName=[SCOPE_DATA.time,SCOPE_DATA.signals(4).values(:,1:2)]  SampleTime=SAMPLING_TIME
  Output16 : FromWorkspace  VariableName=[SCOPE_DATA.time,SCOPE_DATA.signals(3).values(:,1:2)]  SampleTime=SAMPLING_TIME
  Output18 : FromWorkspace  VariableName=[SCOPE_DATA.time,SCOPE_DATA.signals(2).values(:,1:2)]  SampleTime=SAMPLING_TIME
  Output2 : FromWorkspace  VariableName=[SCOPE_DATA.time,SCOPE_DATA.signals(10).values]  SampleTime=SAMPLING_TIME
  Output20 : FromWorkspace  VariableName=[SCOPE_DATA.time,SCOPE_DATA.signals(1).values(:,1:2)]  SampleTime=SAMPLING_TIME
  Output23 : FromWorkspace  VariableName=[SCOPE_DATA.time,SCOPE_DATA.signals(7).values(:,1:4)]  SampleTime=SAMPLING_TIME
  Output24 : FromWorkspace  VariableName=[SCOPE_DATA.time,SCOPE_DATA.signals(8).values(:,1:4)]  SampleTime=SAMPLING_TIME
  Output3 : FromWorkspace  VariableName=[SCOPE_DATA.time,SCOPE_DATA.signals(5).values(:,3)]  SampleTime=SAMPLING_TIME
  Output4 : FromWorkspace  VariableName=[SCOPE_DATA.time,SCOPE_DATA.signals(5).values(:,1:2)]  SampleTime=SAMPLING_TIME
  Output5 : FromWorkspace  VariableName=[SCOPE_DATA.time,SCOPE_DATA.signals(12).values(:,1:2)]  SampleTime=SAMPLING_TIME
  Output6 : FromWorkspace  VariableName=[SCOPE_DATA.time,SCOPE_DATA.signals(11).values(:,1)]  SampleTime=SAMPLING_TIME
  Output7 : FromWorkspace  VariableName=[SCOPE_DATA.time,SCOPE_DATA.signals(6).values(:,1:2)]  SampleTime=SAMPLING_TIME
  SCOPE_TEST : Scope  NumInputPorts=12
  wires:
  Output16/1 -> Gain8/1
  Output23/1 -> Demux/1
  Demux/1 -> [Y5_REF_T]
  Output4/1 -> Demux2/1
  Demux3/1 -> [Y4_REF_T]
  Demux4/1 -> [Y3_REF_T]
  Demux5/1 -> [Y2_REF_T]
  Demux6/1 -> [Y1_REF_T]
  Output20/1 -> Demux6/1
  Output18/1 -> Demux5/1
  Gain8/1 -> Demux4/1
  Output14/1 -> Demux3/1
  Output7/1 -> Demux12/1
  Output24/1 -> Demux1/1
  Demux1/1 -> [Y7_REF_T]
  [U4_T] -> Mux1/2
  [U3_T] -> Mux1/1
  [Y6_REF_T] -> Mux2/2
  [Y5_REF_T] -> Mux2/1
  [Y7_REF_T] -> Mux3/1
  [Y8_REF_T] -> Mux3/2
  Mux3/1 -> Data Store Write1/7
  Demux14/2 -> [Y6_S]
  Demux14/1 -> [Y5_S]
  Demux16/1 -> [Y7_S]
  Demux9/1 -> [U1_S]
  Demux18/2 -> [MR4_S]
  Demux17/1 -> [MR1_S]
  Demux10/2 -> [U4_S]
  Demux9/2 -> [U2_S]
  Demux18/1 -> [MR3_S]
  Demux10/1 -> [U3_S]
  Demux17/2 -> [MR2_S]
  Demux16/2 -> [Y8_S]
  Data Store Read2/1 -> [Y1_S]
  Data Store Read2/2 -> [Y2_S]
  Data Store Read2/3 -> [Y3_S]
  Data Store Read2/4 -> [Y4_S]
  Data Store Read2/9 -> Demux17/1
  Data Store Read2/10 -> Demux18/1
  Gain1/1 -> SCOPE_TEST/3
  Mux8/1 -> SCOPE_TEST/5
  Mux12/1 -> SCOPE_TEST/4
  [Y4_S] -> Mux12/2
  [U1_S] -> Mux8/1
  [U2_S] -> Mux8/2
  Mux6/1 -> SCOPE_TEST/1
  Mux4/1 -> SCOPE_TEST/2
  [Y3_S] -> Mux7/2
  Mux7/1 -> Gain1/1
  Mux14/1 -> SCOPE_TEST/6
  [U4_S] -> Mux14/2
  [U3_S] -> Mux14/1
  Mux9/1 -> SCOPE_TEST/7
  Mux15/1 -> SCOPE_TEST/8
  [MR4_S] -> Mux10/2
  [MR2_S] -> Mux11/2
  [MR1_S] -> Mux11/1
  [MR3_S] -> Mux10/1
  Mux10/1 -> SCOPE_TEST/10
  Mux11/1 -> SCOPE_TEST/9
  Mux2/1 -> Data Store Write1/6
  [MR4_T] -> Delay19/1
  [MR3_T] -> Delay18/1
  [MR2_T] -> Mux11/4
  [MR1_T] -> Mux11/3
  [Y7_REF_T] -> Mux15/1
  [Y5_REF_T] -> Delay14/1
  [U4_T] -> Delay13/1
  [U3_T] -> Delay12/1
  [U2_T] -> Delay10/1
  [U1_T] -> Delay9/1
  [Y4_T] -> Delay8/1
  [Y4_REF_T] -> Delay7/1
  [Y3_T] -> Delay6/1
  [Y3_REF_T] -> Delay5/1
  Data Store Read2/5 -> Demux9/1
  Data Store Read2/6 -> Demux10/1
  Data Store Read2/7 -> Demux14/1
  Data Store Read2/8 -> Demux16/1
  [Y1_REF_T] -> Data Store Write1/2
  [Y2_REF_T] -> Data Store Write1/3
  [Y4_REF_T] -> Data Store Write1/5
  [Y3_REF_T] -> Data Store Write1/4
  Output1/1 -> Demux7/1
  Output2/1 -> Demux8/1
  [Y1_S] -> Mux6/2
  [Y2_S] -> Mux4/2
  [Y1_REF_T] -> Delay1/1
  [Y1_T] -> Delay2/1
  [Y2_REF_T] -> Delay3/1
  [Y2_T] -> Delay4/1
  Mux1/1 -> Data Store Write1/1
  [BATT_VOLT] -> Data Store Write1/8
  [BATT_VOLT] -> Delay11/1
  Demux6/2 -> [Y1_T]
  Demux5/2 -> [Y2_T]
  Demux4/2 -> [Y3_T]
  Demux3/2 -> [Y4_T]
  Demux2/1 -> [U1_T]
  Demux12/1 -> [U3_T]
  Demux12/2 -> [U4_T]
  Demux/3 -> [Y5_T]
  Demux1/4 -> [Y8_T]
  Demux7/1 -> [MR1_T]
  Demux7/2 -> [MR2_T]
  Demux8/1 -> [MR3_T]
  Demux8/2 -> [MR4_T]
  Demux11/1 -> [Y9_REF_T]
  Output5/1 -> Gain4/1
  Gain4/1 -> Demux11/1
  [Y9_T] -> Delay22/1
  [Y9_REF_T] -> Delay21/1
  Mux16/1 -> SCOPE_TEST/11
  [DY9_S] -> Mux16/1
  [DY9_T] -> Delay20/1
  Gain11/1 -> SCOPE_TEST/12
  [Y9_S] -> Mux5/2
  Mux5/1 -> Gain11/1
  Output3/1 -> [BATT_VOLT]
  Output6/1 -> [DY9_T]
  Demux11/2 -> [Y9_T]
  Data Store Read2/11 -> [DY9_S]
  Data Store Read2/12 -> [Y9_S]
  Demux/4 -> [Y6_T]
  Demux1/3 -> [Y7_T]
  Demux/2 -> [Y6_REF_T]
  Demux1/2 -> [Y8_REF_T]
  [Y6_REF_T] -> Delay15/1
  [Y5_S] -> Mux9/3
  [Y6_S] -> Mux9/4
  [Y5_T] -> Delay16/1
  [Y6_T] -> Delay17/1
  [Y8_REF_T] -> Mux15/2
  [Y7_S] -> Mux15/3
  [Y8_S] -> Mux15/4
  [Y7_T] -> Mux15/5
  [Y8_T] -> Mux15/6
  Demux2/2 -> [U2_T]
  Delay1/1 -> Mux6/1
  Delay2/1 -> Mux6/3
  Delay3/1 -> Mux4/1
  Delay4/1 -> Mux4/3
  Delay5/1 -> Mux7/1
  Delay6/1 -> Mux7/3
  Delay7/1 -> Mux12/1
  Delay8/1 -> Mux12/3
  Delay9/1 -> Mux8/3
  Delay10/1 -> Mux8/4
  Delay11/1 -> Mux8/5
  Delay12/1 -> Mux14/3
  Delay13/1 -> Mux14/4
  Delay14/1 -> Mux9/1
  Delay15/1 -> Mux9/2
  Delay16/1 -> Mux9/5
  Delay17/1 -> Mux9/6
  Delay18/1 -> Mux10/3
  Delay19/1 -> Mux10/4
  Delay20/1 -> Mux16/2
  Delay21/1 -> Mux5/1
  Delay22/1 -> Mux5/3

== system CAR_CONTROL_SYSTEM/NAVIGATION/MPC CONTROL FOR NAVIGATION VELOCITY MAGNITUDE AND ANGLE ==
  Input : Inport  OutDataTypeStr=Bus: CONTROL_Bus
  Enable : EnablePort
  Bus Selector : BusSelector  OutputSignals=INPUT.NAV_MO,TARGET.NAV_REF,PARAM.NAV_MPC.OV_WEIGHTS,PARAM.NAV_MPC.MVR_WEIGHTS,PARAM.NAV_MPC.PRED_HRZ,PARAM.NAV_MPC.CTRL_HRZ,TARGET.NAV_REF_MPC
  Compare To Constant : simulink/Logic and Bit Operations/Compare To Constant  relop===  const=3  OutDataTypeStr=boolean
  Constant1 : Constant  Value=CONTROL_INI.STATE.CONTROL_MODE  OutDataTypeStr=single  SampleTime=CONTROL_INI.PARAM.NAV_MPC.SAMPLING_TIME
  Gain1 : Gain  Gain=ones(1,CONTROL_INI.PARAM.NAV_MPC.PRED_HRZ)  Multiplication=Matrix(u*K)  OutDataTypeStr=double
  MPC Controller : mpclib/MPC Controller  SCDEnableBlockLinearizationSpecification=on  mpcobj=NAV_MPC_CONTROL  x0=mpcstate(NAV_MPC_CONTROL)  is_multiple=0  enable_value=0  return_u0=off  updateMPCinCallerWorkspace=on  md_inport=off  mv_inport=off  uref_inport=off  return_cost=off  return_mvseq=off  return_qpstatus=off  return_xseq=off  return_state=off  return_ovseq=off  state_inport=off  umin_inport=off  umax_inport=off  ymin_inport=off  ymax_inport=off  cc_inport=off  ywt_inport=on  uwt_inport=off  duwt_inport=on  rhoeps_inport=off  pm_inport=on  MaximumP=50  HorizonChoice=VariableHorizon  n_ts=1  n_p=50  n_mv=2  n_md=0  n_ud=0  n_mo=2  n_uo=0  BlockDataType=double  SampleTimeInherited=off  switch_inport=off
  MVR WEIGHTS : Display
  OV WEIGHTS : Display
  Switch : Switch  Criteria=u2 > Threshold  Threshold=0.5  SaturateOnIntegerOverflow=off  InputSameDT=off
  Transpose : Math  Operator=transpose  SignedPower=on
  Transpose1 : Math  Operator=transpose  SignedPower=on
  Output : Outport
  wires:
  Bus Selector/4 -> MPC Controller/4, MVR WEIGHTS/1  "<MVR_WEIGHTS>"
  Bus Selector/5 -> MPC Controller/5  "<PRED_HRZ>"
  Bus Selector/6 -> Transpose/1  "<CTRL_HRZ>"
  Transpose/1 -> MPC Controller/6
  Bus Selector/2 -> Gain1/1  "<NAV_REF>"
  Bus Selector/1 -> MPC Controller/1  "<NAV_MO>"
  Switch/1 -> MPC Controller/2
  Bus Selector/7 -> [TGT_LA]  "<NAV_REF_MPC>"
  Compare To Constant/1 -> Switch/2
  Constant1/1 -> Compare To Constant/1
  Gain1/1 -> Transpose1/1
  [TGT_LA] -> Switch/1
  Transpose1/1 -> Switch/3
  Input/1 -> Bus Selector/1
  Bus Selector/3 -> MPC Controller/3, OV WEIGHTS/1  "<OV_WEIGHTS>"
  MPC Controller/1 -> Output/1

== system CAR_CONTROL_SYSTEM/NAVIGATION/NAVIGATION TARGETS ==
  Enable : EnablePort
  Data Store Read7 : DataStoreRead  DataStoreName=CONTROL  SampleTime=SAMPLING_TIME  IndexOptions=Index vector (dialog)  Indices=1  OutputSizes=1
  Data Store Write : DataStoreWrite  DataStoreName=CONTROL  SampleTime=SAMPLING_TIME  IndexOptions=Index vector (dialog)  Indices=1  OutputSizes=1
  TRAJECTORY PLANNER (POLYNOMIAL IN Vx & Vy) : MATLAB Function  Priority=10  TreatAsAtomicUnit=on
  wires:
  Data Store Read7/1 -> TRAJECTORY PLANNER (POLYNOMIAL IN Vx & Vy)/1(CONTROL_IN)
  TRAJECTORY PLANNER (POLYNOMIAL IN Vx & Vy)/1(CONTROL) -> Data Store Write/1

== system CAR_CONTROL_SYSTEM/SIMULATION/ACCELERATION RATE ==
  CONTROL MOTOR VOLT : Inport
  MOTOR VOLT MAX : Inport  Port=2
  Gain : Gain  Gain=10/MD25.PWM_MAX/25e-3*SAMPLING_TIME
  Gain2 : Gain  Gain=-1
  Gain3 : Gain  Gain=-1
  Quantizer : Quantizer  QuantizationInterval=CONTROL_INI.PARAM.MOTOR_VOLT_MAX(1)/127
  Saturation Dynamic : simulink/Discontinuities/Saturation Dynamic  OutMin=[]  OutMax=[]  OutDataTypeStr=Inherit: Same as second input  OutDataType=fixdt(1, 16)  OutScaling=2^-10  DoSatur=off
  Saturation Dynamic1 : simulink/Discontinuities/Saturation Dynamic  OutMin=[]  OutMax=[]  OutDataTypeStr=Inherit: Same as second input  OutDataType=fixdt(1, 16)  OutScaling=2^-10  DoSatur=off
  Sum : Sum  Inputs=|+-
  Sum1 : Sum  Inputs=|++
  Unit Delay : UnitDelay  SampleTime=-1  HasFrameUpgradeWarning=on
  REAL MOTOR VOLT : Outport
  wires:
  Gain3/1 -> Saturation Dynamic1/3
  Gain2/1 -> Saturation Dynamic/3
  Sum/1 -> Saturation Dynamic/2
  MOTOR VOLT MAX/1 -> Gain/1, Gain3/1, Saturation Dynamic1/1
  Sum1/1 -> Saturation Dynamic1/2
  Gain/1 -> Gain2/1, Saturation Dynamic/1
  Saturation Dynamic/1 -> Sum1/1
  Saturation Dynamic1/1 -> REAL MOTOR VOLT/1, Unit Delay/1
  Unit Delay/1 -> Sum/2, Sum1/2
  CONTROL MOTOR VOLT/1 -> Quantizer/1
  Quantizer/1 -> Sum/1

== system CAR_CONTROL_SYSTEM/SIMULATION/CIRCUIT ==
  xA : Inport  SampleTime=ts
  yA : Inport  Port=2  SampleTime=ts
  theta (rad) : Inport  Port=3  SampleTime=ts
  Enable : EnablePort
  CIRCUITO : MATLAB Function  TreatAsAtomicUnit=on
  Constant2 : Constant  Value=param  SampleTime=ts
  Data Type Conversion : DataTypeConversion  OutDataTypeStr=double  SaturateOnIntegerOverflow=off  RndMeth=Floor
  Mux : Mux  Inputs=2
  Unit Delay : UnitDelay  InitialCondition=1  SampleTime=MODEL_INI.PARAM.SIM_SAMPLING_TIME  HasFrameUpgradeWarning=on
  dist (mm) : Outport  VectorParamsAs1DForOutWhenUnconnected=off
  theta_circ (rad) : Outport  Port=2  VectorParamsAs1DForOutWhenUnconnected=off
  d_sens (m) : Outport  Port=3  VectorParamsAs1DForOutWhenUnconnected=off
  rampa : Outport  Port=4  VectorParamsAs1DForOutWhenUnconnected=off
  estado : Outport  Port=5  VectorParamsAs1DForOutWhenUnconnected=off
  wires:
  xA/1 -> CIRCUITO/1(xi)
  yA/1 -> CIRCUITO/2(yi)
  CIRCUITO/1(d) -> dist (mm)/1
  CIRCUITO/2(theta_circ) -> theta_circ (rad)/1
  CIRCUITO/5(rampa) -> rampa/1
  Constant2/1 -> Data Type Conversion/1
  CIRCUITO/6(estado) -> estado/1, Unit Delay/1
  Unit Delay/1 -> CIRCUITO/5(est_ant)
  theta (rad)/1 -> CIRCUITO/3(theta)
  CIRCUITO/4(d2) -> Mux/2
  CIRCUITO/3(d1) -> Mux/1
  Mux/1 -> d_sens (m)/1  "m"
  Data Type Conversion/1 -> CIRCUITO/4(param)

== system CAR_CONTROL_SYSTEM/SIMULATION/MCS DELAY ==
  CONTROL_IN : Inport
  Bus Assignment2 : BusAssignment  AssignedSignals=INPUT.MCS_EULER_ANG,INPUT.MCS_EARTH_POS
  Bus Selector1 : BusSelector  OutputSignals=INPUT.MCS_EULER_ANG,INPUT.MCS_EARTH_POS
  MCS_DELAY : Delay  DelayLength=round(CONTROL_INI.PARAM.MCS_DELAY/SAMPLING_TIME)
  "MCS_DELAY " : Delay  DelayLength=round(CONTROL_INI.PARAM.MCS_DELAY/SAMPLING_TIME)
  Scope : Scope
  Scope1 : Scope
  CONTROL_OUT : Outport  OutDataTypeStr=Bus: CONTROL_Bus
  wires:
  "MCS_DELAY "/1 -> Scope1/1, Bus Assignment2/3
  MCS_DELAY/1 -> Bus Assignment2/2
  Bus Selector1/2 -> Scope/1, "MCS_DELAY "/1  "<MCS_EARTH_POS>"
  Bus Selector1/1 -> MCS_DELAY/1  "<MCS_EULER_ANG>"
  CONTROL_IN/1 -> Bus Selector1/1, Bus Assignment2/1
  Bus Assignment2/1 -> CONTROL_OUT/1

== system CAR_CONTROL_SYSTEM/SIMULATION/MOTOR DELAY ==
  Compare To Constant4 : simulink/Logic and Bit Operations/Compare To Constant  relop===  const=2  OutDataTypeStr=boolean
  Data Store Read1 : DataStoreRead  DataStoreName=CONTROL  SampleTime=SAMPLING_TIME  DataStoreElements=CONTROL.PARAM.SAMPLING_TIME  IndexOptions=Index vector (dialog)  Indices=1  OutputSizes=1
  Data Store Read17 : DataStoreRead  DataStoreName=CONTROL  SampleTime=SAMPLING_TIME  DataStoreElements=CONTROL.STATE.MOTOR_DELAY_MODE  IndexOptions=Index vector (dialog)  Indices=1  OutputSizes=1
  Data Store Read3 : DataStoreRead  DataStoreName=CONTROL  SampleTime=SAMPLING_TIME  DataStoreElements=CONTROL.OUTPUT.MOTOR_VOLT(:,:)  IndexOptions=Index vector (dialog)  Indices=1  OutputSizes=1
  Data Store Read6 : DataStoreRead  DataStoreName=CONTROL  SampleTime=SAMPLING_TIME  DataStoreElements=CONTROL.PARAM.MOTOR_DELAY  IndexOptions=Index vector (dialog)  Indices=1  OutputSizes=1
  Data Store Read7 : DataStoreRead  DataStoreName=CONTROL  SampleTime=SAMPLING_TIME  DataStoreElements=CONTROL.OUTPUT.MOTOR_VOLT_CD(:,:)  IndexOptions=Index vector (dialog)  Indices=1  OutputSizes=1
  Data Store Write1 : DataStoreWrite  DataStoreName=CONTROL  DataStoreElements=CONTROL.OUTPUT.MOTOR_VOLT_CD(:,:)  IndexOptions=Index vector (dialog)  Indices=1  OutputSizes=1
  Data Store Write4 : DataStoreWrite  DataStoreName=CONTROL  DataStoreElements=CONTROL.OUTPUT.MOTOR_VOLT(:,:)  IndexOptions=Index vector (dialog)  Indices=1  OutputSizes=1
  Data Type Conversion : DataTypeConversion  OutDataTypeStr=double  SaturateOnIntegerOverflow=off  RndMeth=Floor
  Delay : Delay  DelayLengthSource=Input port  DelayLengthUpperLimit=20  SampleTime=SAMPLING_TIME
      settings: InputPortMap=u0,p1
  Delay2 : Delay  DelayLengthSource=Input port  DelayLengthUpperLimit=20  SampleTime=SAMPLING_TIME
      settings: InputPortMap=u0,p1
  Product : Product  Inputs=*/*
  Rounding Function : Rounding
  wires:
  Data Store Read3/1 -> Delay/1
  Delay/1 -> Data Store Write4/1
  Rounding Function/1 -> Delay2/2, Delay/2
  Product/1 -> Rounding Function/1
  Data Store Read1/1 -> Product/2
  Data Store Read6/1 -> Product/1
  Data Store Read7/1 -> Delay2/1
  Delay2/1 -> Data Store Write1/1
  Data Store Read17/1 -> Compare To Constant4/1
  Data Type Conversion/1 -> Product/3
  Compare To Constant4/1 -> Data Type Conversion/1

== system CAR_CONTROL_SYSTEM/SIMULATION/RAMP1 ==
  Constant : Constant  Value=MODEL_INI.PARAM.SIM_SAMPLING_TIME  SampleTime=MODEL_INI.PARAM.SIM_SAMPLING_TIME
  Constant1 : Constant  Value=0  SampleTime=MODEL_INI.PARAM.SIM_SAMPLING_TIME
  Constant2 : Constant  Value=MODEL_INI.CIRCUIT.CURVE_RADIUS  SampleTime=MODEL_INI.PARAM.SIM_SAMPLING_TIME
  Constant3 : Constant  Value=pi*MODEL_INI.CIRCUIT.CURVE_RADIUS  SampleTime=MODEL_INI.PARAM.SIM_SAMPLING_TIME
  Data Store Read3 : DataStoreRead  DataStoreName=MODEL  SampleTime=MODEL_INI.PARAM.SIM_SAMPLING_TIME  DataStoreElements=MODEL.OUTPUT.FORWARD_VEL  IndexOptions=Index vector (dialog)  Indices=1  OutputSizes=1
  Discrete Filter : DiscreteFilter  Numerator=[1-0.995]  Denominator=[1 -0.995]
  Divide : Product  Inputs=*/
  Divide1 : Product  Inputs=*/
  Gain : Gain  Gain=-1
  Logical Operator1 : Logic  AllPortsSameDT=off  OutDataTypeStr=boolean
  Math Function : Math  Operator=rem
  OFFSET : Constant  Value=20  SampleTime=MODEL_INI.PARAM.SIM_SAMPLING_TIME
  PERIOD : Constant  Value=40  SampleTime=MODEL_INI.PARAM.SIM_SAMPLING_TIME
  Relational Operator : RelationalOperator  Operator=<=  OutDataTypeStr=boolean  RndMeth=Simplest  InputSameDT=off
  Relational Operator1 : RelationalOperator  OutDataTypeStr=boolean  RndMeth=Simplest  InputSameDT=off
  Sum : Sum  Inputs=|++
  Sum1 : Sum  Inputs=++|
  Switch1 : Switch  Criteria=u2 > Threshold  Threshold=0.5  SaturateOnIntegerOverflow=off  InputSameDT=off
  Unit Delay : UnitDelay  SampleTime=-1  HasFrameUpgradeWarning=on
  WALL RATE : Outport  VectorParamsAs1DForOutWhenUnconnected=off
  wires:
  Unit Delay/1 -> Sum/2, Math Function/1  "TIME (s)"
  Sum/1 -> Unit Delay/1
  Constant/1 -> Sum/1
  Constant1/1 -> Switch1/3
  PERIOD/1 -> Math Function/2
  Math Function/1 -> Relational Operator/1, Relational Operator1/1
  OFFSET/1 -> Relational Operator1/2, Sum1/1
  Relational Operator1/1 -> Logical Operator1/1
  Relational Operator/1 -> Logical Operator1/2
  Logical Operator1/1 -> Switch1/2
  Switch1/1 -> Gain/1
  Divide/1 -> Switch1/1
  Data Store Read3/1 -> Discrete Filter/1
  Constant2/1 -> Divide/2
  Sum1/1 -> Relational Operator/2
  Constant3/1 -> Divide1/1
  Divide1/1 -> Sum1/2
  Gain/1 -> WALL RATE/1
  Discrete Filter/1 -> Divide/1, Divide1/2

== system CAR_CONTROL_SYSTEM/SIMULATION/RANGE NOISE ==
  Matrix Concatenate1 : Concatenate  Mode=Multidimensional array  ConcatenateDimension=2
  RANGE_DIST_FRONT : RandomNumber  Seed=10000  SampleTime=SAMPLING_TIME
  RANGE_DIST_REAR : RandomNumber  Seed=11000  SampleTime=SAMPLING_TIME
  WFL_NOISE : Outport  VectorParamsAs1DForOutWhenUnconnected=off
  wires:
  RANGE_DIST_FRONT/1 -> Matrix Concatenate1/1
  RANGE_DIST_REAR/1 -> Matrix Concatenate1/2
  Matrix Concatenate1/1 -> WFL_NOISE/1

== system CAR_CONTROL_SYSTEM/SIMULATION/RC TRANSMITTER  ==
  note: SWB: CH2 y CH3
  note: SWC: CH4 y CH5
  BUS UPDATE : MATLAB Function  Priority=20  TreatAsAtomicUnit=on
  Bias{,1..3} (4 alike) : Bias  Bias=1500  SaturateOnIntegerOverflow=off
  Bus Selector : BusSelector  OutputSignals=TARGET.RC_CH_PU
  Constant5 : Constant  Value=zeros(8,1)  SampleTime=-1
  Data Store Read19 : DataStoreRead  DataStoreName=CONTROL  SampleTime=SAMPLING_TIME  IndexOptions=Index vector (dialog)  Indices=1  OutputSizes=1
  Data Store Write1 : DataStoreWrite  DataStoreName=CONTROL  IndexOptions=Index vector (dialog)  Indices=1  OutputSizes=1
  Data Type Conversion : DataTypeConversion  OutDataTypeStr=double  SaturateOnIntegerOverflow=off  RndMeth=Floor
  Demux : Demux  Outputs=[1 1 1 1 -1]
  Demux1 : Demux  Outputs=[1 1 1 1 1 -1]
  Display{,1..3} (4 alike) : Display
  Gain{1..4} (4 alike) : Gain  Gain=500
  Joystick Input : vrlib/Joystick Input  joyid=1  adjustports=on  forcefeed=off
  Mux : Mux  Inputs=7
  Rate Transition : RateTransition  OutPortSampleTime=SAMPLING_TIME
  Rate Transition1 : RateTransition  OutPortSampleTime=SAMPLING_TIME
  SWB : Subsystem
  SWC : Subsystem
  Saturation{,1..3} (4 alike) : Saturate  UpperLimit=1  LowerLimit=-1
  Terminator : Terminator
  Terminator1 : Terminator
  Terminator2 : Terminator
  wires:
  Gain1/1 -> Bias/1
  Saturation/1 -> Gain1/1
  Joystick Input/1 -> Rate Transition/1
  Joystick Input/2 -> Rate Transition1/1
  Gain2/1 -> Bias1/1
  Saturation1/1 -> Gain2/1
  Demux/1 -> Saturation/1
  Demux/2 -> Saturation1/1
  Saturation3/1 -> Gain4/1
  Gain4/1 -> Bias3/1
  Saturation2/1 -> Gain3/1
  Gain3/1 -> Bias2/1
  Demux/3 -> Saturation2/1
  Demux/4 -> Saturation3/1
  Demux/5 -> Terminator/1
  Bias/1 -> Mux/1  "RC_CH1_RAW (ROLL)"
  Bias1/1 -> Mux/2
  Bias2/1 -> Mux/3  "RC_CH1_RAW (ROLL)"
  Bias3/1 -> Mux/4
  Data Store Read19/1 -> BUS UPDATE/1(CONTROL_IN)
  Mux/1 -> BUS UPDATE/2(CH_RAW), Display2/1
  BUS UPDATE/1(CONTROL) -> Data Store Write1/1, Bus Selector/1
  Rate Transition/1 -> Display/1, Demux/1
  Rate Transition1/1 -> Data Type Conversion/1, Display1/1
  Bus Selector/1 -> Display3/1  "<RC_CH_PU>"
  Constant5/1 -> Mux/7
  Demux1/1 -> Terminator1/1
  Demux1/6 -> Terminator2/1
  Data Type Conversion/1 -> Demux1/1
  Demux1/2 -> SWB/1(UP)
  Demux1/3 -> SWB/2(DOWN)
  Demux1/4 -> SWC/1(UP)
  Demux1/5 -> SWC/2(DOWN)
  SWB/1(SWITCH) -> Mux/5
  SWC/1(SWITCH) -> Mux/6

== system CAR_CONTROL_SYSTEM/SIMULATION/READ ENCODER ==
  Data Store Read10 : DataStoreRead  Priority=30  DataStoreName=MODEL  SampleTime=SAMPLING_TIME  IndexOptions=Index vector (dialog)  Indices=1  OutputSizes=1
  Data Store Read4 : DataStoreRead  DataStoreName=CONTROL  SampleTime=SAMPLING_TIME  IndexOptions=Index vector (dialog)  Indices=1  OutputSizes=1
  Data Store Write2 : DataStoreWrite  DataStoreName=CONTROL  IndexOptions=Index vector (dialog)  Indices=1  OutputSizes=1
  READ_ENCODER : MATLAB Function  TreatAsAtomicUnit=on
  Scope : Scope  NumInputPorts=2
  wires:
  Data Store Read10/1 -> READ_ENCODER/1(MODEL)
  Data Store Read4/1 -> READ_ENCODER/2(CONTROL_IN)
  READ_ENCODER/1(CONTROL) -> Data Store Write2/1
  READ_ENCODER/2(left_enc) -> Scope/1
  READ_ENCODER/3(right_enc) -> Scope/2
